simulink model "Trab1_desafio2"  (R2018a)
settings: Solver=VariableStepAuto  StartTime=0.0  StopTime=10  RelTol=1e-6
values from neighbouring files (symbols this model uses):
  A11 = A_til(1:k,1:k)    [Trab1_desafio_2.m]
  A12 = A_til(1:k,k+1:end)    [Trab1_desafio_2.m]
  A22 = A_til(k+1:end,k+1:end)    [Trab1_desafio_2.m]
  B1 = B_til(1:k,1)    [Trab1_desafio_2.m]
  C1 = C_til(:,1:k)    [Trab1_desafio_2.m]
  C2 = C_til(:,k+1:end)    [Trab1_desafio_2.m]
  z0_c = z0(1:2,1)    [Trab1_desafio_2.m]
  z0_uc = z0(3:4,1)    [Trab1_desafio_2.m]
undefined symbols (not defined in the file or in its folder): calcula_entrada
settings Model: Creator=eric-  LastModifiedBy=eric-

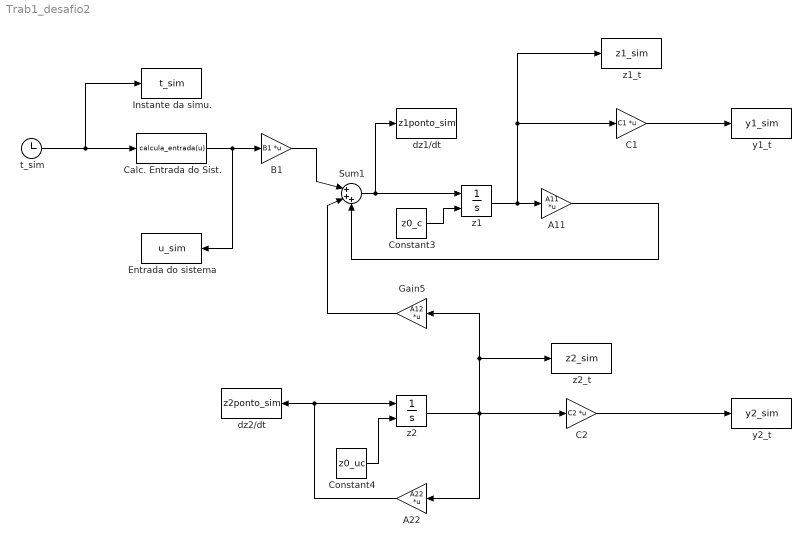
== system Trab1_desafio2 ==
  "A11 " : Gain  Gain=A11  Multiplication=Matrix(K*u)
  A22 : Gain  Gain=A22  Multiplication=Matrix(K*u)
  "B1 " : Gain  Gain=B1  Multiplication=Matrix(K*u)
  C1 : Gain  Gain=C1  Multiplication=Matrix(K*u)
  C2 : Gain  Gain=C2  Multiplication=Matrix(K*u)
  Calc. Entrada do Sist. : MATLABFcn  MATLABFcn=calcula_entrada(u)
  Constant3 : Constant  Value=z0_c
  Constant4 : Constant  Value=z0_uc
  Entrada do sistema : ToWorkspace  VariableName=u_sim  SampleTime=-1
      settings: Save2DSignal=2-D array (concatenate along first dimension)
  Gain5 : Gain  Gain=A12  Multiplication=Matrix(K*u)
  Instante da simu. : ToWorkspace  VariableName=t_sim  SampleTime=-1
      settings: Save2DSignal=2-D array (concatenate along first dimension)
  Sum1 : Sum  Inputs=|+++
  dz1/dt : ToWorkspace  VariableName=z1ponto_sim  SampleTime=-1
      settings: Save2DSignal=2-D array (concatenate along first dimension)
  dz2/dt : ToWorkspace  VariableName=z2ponto_sim  SampleTime=-1
      settings: Save2DSignal=2-D array (concatenate along first dimension)
  t_sim : Clock
  y1_t : ToWorkspace  VariableName=y1_sim  SampleTime=-1
      settings: Save2DSignal=2-D array (concatenate along first dimension)
  y2_t : ToWorkspace  VariableName=y2_sim  SampleTime=-1
      settings: Save2DSignal=2-D array (concatenate along first dimension)
  z1 : Integrator  InitialConditionSource=external  InitialCondition=[3.5;0]
  z1_t : ToWorkspace  VariableName=z1_sim  SampleTime=-1
      settings: Save2DSignal=2-D array (concatenate along first dimension)
  z2 : Integrator  InitialConditionSource=external  InitialCondition=[1;2]
  z2_t : ToWorkspace  VariableName=z2_sim  SampleTime=-1
      settings: Save2DSignal=2-D array (concatenate along first dimension)
  wires:
  Sum1/1 -> dz1/dt/1, z1/1
  "A11 "/1 -> Sum1/3
  "B1 "/1 -> Sum1/1
  Gain5/1 -> Sum1/2
  A22/1 -> dz2/dt/1, z2/1
  z2/1 -> z2_t/1, Gain5/1, C2/1, A22/1
  t_sim/1 -> Calc. Entrada do Sist./1, Instante da simu./1
  Calc. Entrada do Sist./1 -> Entrada do sistema/1, "B1 "/1
  C1/1 -> y1_t/1
  C2/1 -> y2_t/1
  Constant3/1 -> z1/2
  Constant4/1 -> z2/2
  z1/1 -> z1_t/1, C1/1, "A11 "/1
